simulink model "LPDs_single_agent_tech"  (R2023b)
settings: Solver=VariableStepAuto  StartTime=0.0  StopTime=24  FixedStep=0.005  RelTol=1e-6
undefined symbols (not defined in the file): battery_capacity_state_lower_limit, battery_capacity_state_upper_limit, battery_charge_power_state_lower_limit, battery_charge_power_state_upper_limit, battery_discharge_power_state_lower_limit, battery_discharge_power_state_upper_limit, battery_initial_capacity, battery_SOC_state_lower_limit, battery_SOC_state_upper_limit, EV_load_priority_factor, EV_load_rating, EV_load_state_lower_limit, EV_load_state_upper_limit, micro_grid_controller_power_state_lower_limit, micro_grid_controller_power_state_upper_limit, nano_grid_controller_power_rating, nano_grid_controller_power_state_lower_limit, nano_grid_controller_power_state_upper_limit, PV_power_rating, PV_power_state_lower_limit, PV_power_state_upper_limit, static_load_priority_factor, static_load_rating, static_load_state_lower_limit, static_load_state_upper_limit, sum_power_threshold_lower_limit, sum_power_threshold_upper_limit, TCL_load_priority_factor, TCL_load_rating, TCL_load_state_lower_limit, TCL_load_state_upper_limit, Wind_power_rating, Wind_power_state_lower_limit, Wind_power_state_upper_limit
libraries: spsStairGeneratorLib x13, simulink x7, slpidlib x2, rllib x2
(part 3 of 4)

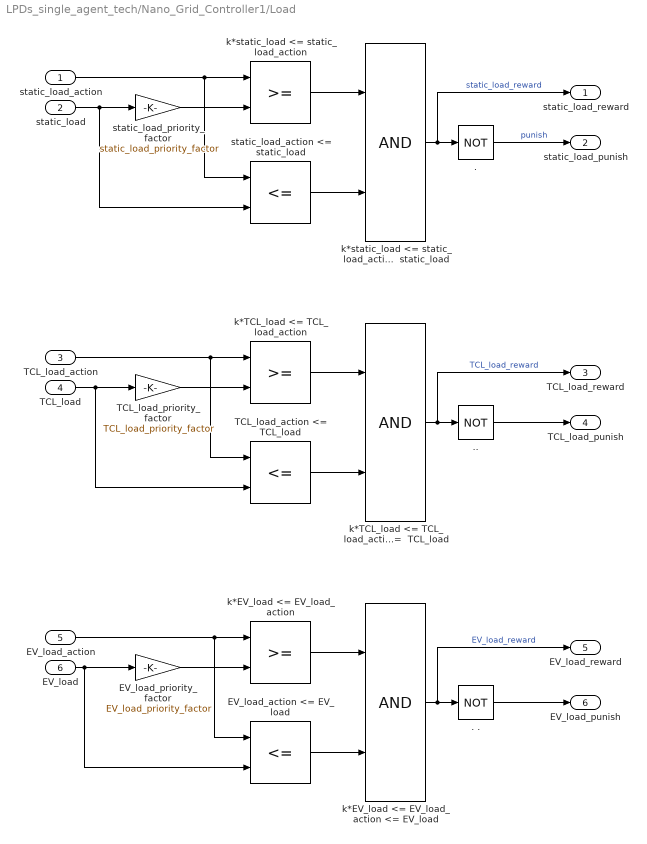
== system LPDs_single_agent_tech/Nano_Grid_Controller1/Load ==
  static_load_action : Inport
  static_load : Inport  Port=2
  TCL_load_action : Inport  Port=3
  TCL_load : Inport  Port=4
  EV_load_action : Inport  Port=5
  EV_load : Inport  Port=6
  . : Logic  Operator=NOT  IconShape=distinctive  AllPortsSameDT=off  OutDataTypeStr=boolean
  . . : Logic  Operator=NOT  IconShape=distinctive  AllPortsSameDT=off  OutDataTypeStr=boolean
  .. : Logic  Operator=NOT  IconShape=distinctive  AllPortsSameDT=off  OutDataTypeStr=boolean
  EV_load_action <= EV_load : RelationalOperator  Operator=<=  OutDataTypeStr=boolean  RndMeth=Simplest  InputSameDT=off
  EV_load_priority_factor : Gain  Gain=EV_load_priority_factor
  TCL_load_action <= TCL_load : RelationalOperator  Operator=<=  OutDataTypeStr=boolean  RndMeth=Simplest  InputSameDT=off
  TCL_load_priority_factor : Gain  Gain=TCL_load_priority_factor
  k*EV_load <= EV_load_action : RelationalOperator  OutDataTypeStr=boolean  RndMeth=Simplest  InputSameDT=off
  k*EV_load <= EV_load_action <= EV_load : Logic  IconShape=distinctive  AllPortsSameDT=off  OutDataTypeStr=boolean
  k*TCL_load <= TCL_load_action : RelationalOperator  OutDataTypeStr=boolean  RndMeth=Simplest  InputSameDT=off
  k*TCL_load <= TCL_load_action <=  TCL_load : Logic  IconShape=distinctive  AllPortsSameDT=off  OutDataTypeStr=boolean
  k*static_load <= static_load_action : RelationalOperator  OutDataTypeStr=boolean  RndMeth=Simplest  InputSameDT=off
  "k*static_load <= static_load_action <=  static_load " : Logic  IconShape=distinctive  AllPortsSameDT=off  OutDataTypeStr=boolean
  static_load_action <= static_load : RelationalOperator  Operator=<=  OutDataTypeStr=boolean  RndMeth=Simplest  InputSameDT=off
  static_load_priority_factor : Gain  Gain=static_load_priority_factor
  static_load_reward : Outport
  static_load_punish : Outport  Port=2
  TCL_load_reward : Outport  Port=3
  TCL_load_punish : Outport  Port=4
  EV_load_reward : Outport  Port=5
  EV_load_punish : Outport  Port=6
  wires:
  "k*static_load <= static_load_action <=  static_load "/1 -> static_load_reward/1, ./1  "static_load_reward"
  EV_load_priority_factor/1 -> k*EV_load <= EV_load_action/2
  EV_load_action <= EV_load/1 -> k*EV_load <= EV_load_action <= EV_load/2
  k*static_load <= static_load_action/1 -> "k*static_load <= static_load_action <=  static_load "/1
  k*TCL_load <= TCL_load_action <=  TCL_load/1 -> TCL_load_reward/1, ../1  "TCL_load_reward"
  k*EV_load <= EV_load_action <= EV_load/1 -> EV_load_reward/1, . ./1  "EV_load_reward"
  k*TCL_load <= TCL_load_action/1 -> k*TCL_load <= TCL_load_action <=  TCL_load/1
  static_load_action <= static_load/1 -> "k*static_load <= static_load_action <=  static_load "/2
  TCL_load_action <= TCL_load/1 -> k*TCL_load <= TCL_load_action <=  TCL_load/2
  EV_load_action/1 -> EV_load_action <= EV_load/1, k*EV_load <= EV_load_action/1
  static_load_priority_factor/1 -> k*static_load <= static_load_action/2
  TCL_load_priority_factor/1 -> k*TCL_load <= TCL_load_action/2
  k*EV_load <= EV_load_action/1 -> k*EV_load <= EV_load_action <= EV_load/1
  TCL_load/1 -> TCL_load_action <= TCL_load/2, TCL_load_priority_factor/1
  TCL_load_action/1 -> k*TCL_load <= TCL_load_action/1, TCL_load_action <= TCL_load/1
  static_load_action/1 -> k*static_load <= static_load_action/1, static_load_action <= static_load/1
  . ./1 -> EV_load_punish/1
  ../1 -> TCL_load_punish/1
  ./1 -> static_load_punish/1  "punish"
  static_load/1 -> static_load_action <= static_load/2, static_load_priority_factor/1
  EV_load/1 -> EV_load_action <= EV_load/2, EV_load_priority_factor/1

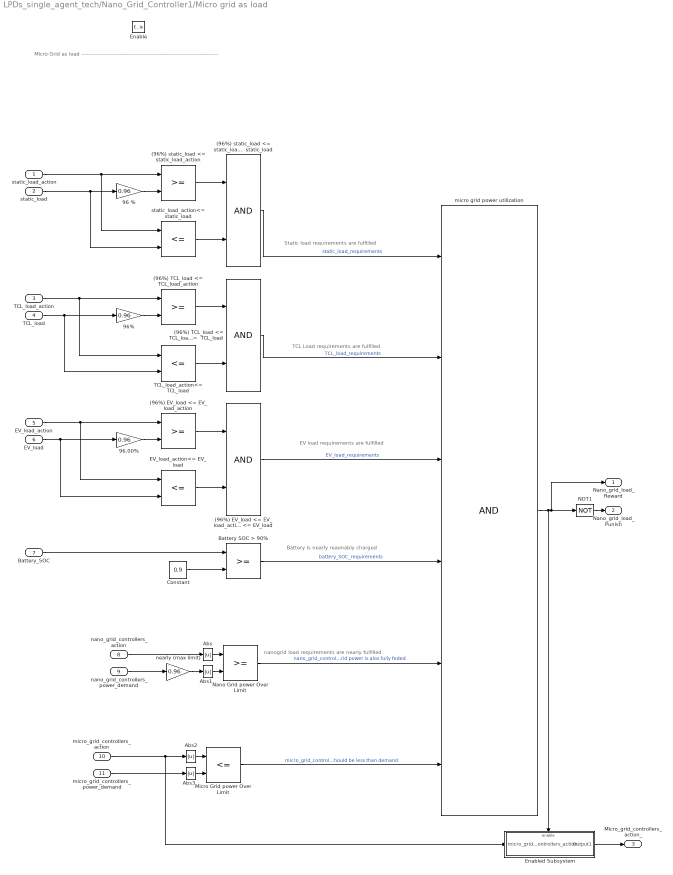
== system LPDs_single_agent_tech/Nano_Grid_Controller1/Micro grid as load ==
  note: Static load requirements are fulfilled
  note: Micro Grid as load
      | ----------------------------------------------------------------------------------
  note: TCL Load requirements are fulfilled
  note: EV load requirements are fulfilled
  note: Battery is nearly reaonably charged
  note: nanogrid load requirements are nearly fulfilled
  static_load_action : Inport
  static_load : Inport  Port=2
  TCL_load_action : Inport  Port=3
  TCL_load : Inport  Port=4
  EV_load_action : Inport  Port=5
  EV_load : Inport  Port=6
  Battery_SOC : Inport  Port=7
  nano_grid_controllers_action : Inport  Port=8
  nano_grid_controllers_power_demand : Inport  Port=9
  micro_grid_controllers_action : Inport  Port=10
  micro_grid_controllers_power_demand : Inport  Port=11
  Enable : EnablePort
  (96%) EV_load <= EV_load_action : RelationalOperator  OutDataTypeStr=boolean  RndMeth=Simplest  InputSameDT=off
  (96%) EV_load <= EV_load_action <= EV_load : Logic  IconShape=distinctive  AllPortsSameDT=off  OutDataTypeStr=boolean
  (96%) TCL_load <= TCL_load_action : RelationalOperator  OutDataTypeStr=boolean  RndMeth=Simplest  InputSameDT=off
  (96%) TCL_load <= TCL_load_action <=  TCL_load : Logic  IconShape=distinctive  AllPortsSameDT=off  OutDataTypeStr=boolean
  (96%) static_load <= static_load_action : RelationalOperator  OutDataTypeStr=boolean  RndMeth=Simplest  InputSameDT=off
  (96%) static_load <= static_load_action <=  static_load : Logic  IconShape=distinctive  AllPortsSameDT=off  OutDataTypeStr=boolean
  96 % : Gain  Gain=0.96
  96% : Gain  Gain=0.96
  96.00% : Gain  Gain=0.96
  Abs{,1..3} (4 alike) : Abs  SaturateOnIntegerOverflow=off
  Battery SOC > 90% : RelationalOperator  OutDataTypeStr=boolean  RndMeth=Simplest  InputSameDT=off
  Constant : Constant  Value=0.9
  EV_load_action<= EV_load : RelationalOperator  Operator=<=  OutDataTypeStr=boolean  RndMeth=Simplest  InputSameDT=off
  Enabled Subsystem : Subsystem  TreatAsAtomicUnit=on
  Micro Grid power Over Limit : RelationalOperator  Operator=<=  OutDataTypeStr=boolean  RndMeth=Simplest  InputSameDT=off
  NOT1 : Logic  Operator=NOT  Inputs=4  IconShape=distinctive  AllPortsSameDT=off  OutDataTypeStr=boolean
  Nano Grid power Over Limit : RelationalOperator  OutDataTypeStr=boolean  RndMeth=Simplest  InputSameDT=off
  TCL_load_action<= TCL_load : RelationalOperator  Operator=<=  OutDataTypeStr=boolean  RndMeth=Simplest  InputSameDT=off
  micro grid power utilization : Logic  Inputs=6  IconShape=distinctive  AllPortsSameDT=off  OutDataTypeStr=boolean
  nearly (max limit) : Gain  Gain=0.96
  static_load_action<= static_load : RelationalOperator  Operator=<=  OutDataTypeStr=boolean  RndMeth=Simplest  InputSameDT=off
  Nano_grid_load_Reward : Outport
  Nano_grid_load_Punish : Outport  Port=2
  Micro_grid_controllers_action_ : Outport  Port=3
  wires:
  (96%) TCL_load <= TCL_load_action <=  TCL_load/1 -> micro grid power utilization/2  "TCL_load_requirements"
  (96%) EV_load <= EV_load_action <= EV_load/1 -> micro grid power utilization/3  "EV_load_requirements"
  96%/1 -> (96%) TCL_load <= TCL_load_action/2
  TCL_load_action<= TCL_load/1 -> (96%) TCL_load <= TCL_load_action <=  TCL_load/2
  (96%) static_load <= static_load_action/1 -> (96%) static_load <= static_load_action <=  static_load/1
  TCL_load_action/1 -> TCL_load_action<= TCL_load/1, (96%) TCL_load <= TCL_load_action/1
  96 %/1 -> (96%) static_load <= static_load_action/2
  96.00%/1 -> (96%) EV_load <= EV_load_action/2
  (96%) EV_load <= EV_load_action/1 -> (96%) EV_load <= EV_load_action <= EV_load/1
  EV_load_action<= EV_load/1 -> (96%) EV_load <= EV_load_action <= EV_load/2
  static_load/1 -> static_load_action<= static_load/2, 96 %/1
  static_load_action<= static_load/1 -> (96%) static_load <= static_load_action <=  static_load/2
  EV_load/1 -> EV_load_action<= EV_load/2, 96.00%/1
  (96%) TCL_load <= TCL_load_action/1 -> (96%) TCL_load <= TCL_load_action <=  TCL_load/1
  Constant/1 -> Battery SOC > 90%/2
  static_load_action/1 -> static_load_action<= static_load/1, (96%) static_load <= static_load_action/1
  Battery SOC > 90%/1 -> micro grid power utilization/4  "battery_SOC_requirements"
  EV_load_action/1 -> EV_load_action<= EV_load/1, (96%) EV_load <= EV_load_action/1
  TCL_load/1 -> TCL_load_action<= TCL_load/2, 96%/1
  Battery_SOC/1 -> Battery SOC > 90%/1
  (96%) static_load <= static_load_action <=  static_load/1 -> micro grid power utilization/1  "static_load_requirements"
  Nano Grid power Over Limit/1 -> micro grid power utilization/5  "nano_grid_controllers_action >= 96% nano_grid_controllers_power_supply nano grid power is alos fully feded"
  nano_grid_controllers_power_demand/1 -> nearly (max limit)/1
  micro grid power utilization/1 -> NOT1/1, Nano_grid_load_Reward/1, Enabled Subsystem/Enable
  Enabled Subsystem/1(Output1) -> Micro_grid_controllers_action_/1
  NOT1/1 -> Nano_grid_load_Punish/1
  nano_grid_controllers_action/1 -> Abs/1
  Abs1/1 -> Nano Grid power Over Limit/2
  Abs/1 -> Nano Grid power Over Limit/1
  nearly (max limit)/1 -> Abs1/1
  Abs3/1 -> Micro Grid power Over Limit/2
  micro_grid_controllers_action/1 -> Enabled Subsystem/1(micro_grid_controllers_action), Abs2/1
  Abs2/1 -> Micro Grid power Over Limit/1
  Micro Grid power Over Limit/1 -> micro grid power utilization/6  "micro_grid_controllers_action >= micro_grid_controllers_power_supply micro grid feeding power should be less than demand"
  micro_grid_controllers_power_demand/1 -> Abs3/1

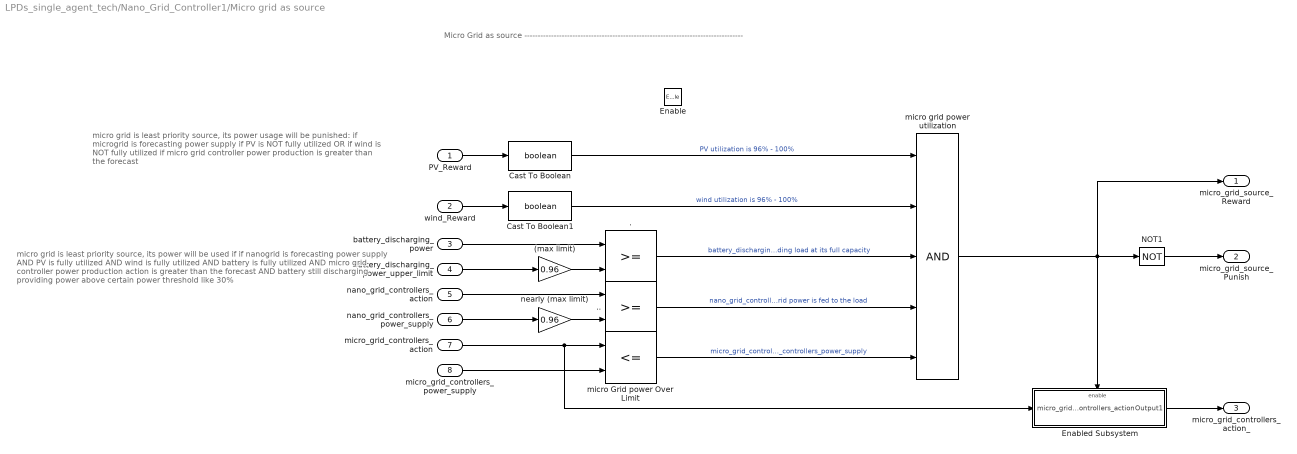
== system LPDs_single_agent_tech/Nano_Grid_Controller1/Micro grid as source ==
  note: Micro Grid as source
      | ----------------------------------------------------------------------------------
  note: micro grid is least priority source, its power usage will be punished:
      | if microgrid is forecasting power supply
      | if PV is NOT fully utilized OR
      | if wind is NOT fully utilized
      | if micro grid controller power production is greater than the forecast
  note: micro grid is least priority source, its power will be used if
      | if nanogrid is forecasting power supply
      | AND
      | PV is fully utilized
      | AND
      | wind is fully utilized
      | AND
      | battery is fully utilized
      | AND
      | micro grid controller power production action is greater than the forecast
      | AND
      | battery still discharging providing power above certain power threshold like 30%
  PV_Reward : Inport
  wind_Reward : Inport  Port=2
  battery_discharging_power : Inport  Port=3
  battery_discharging_power_upper_limit : Inport  Port=4
  nano_grid_controllers_action : Inport  Port=5
  nano_grid_controllers_power_supply : Inport  Port=6
  micro_grid_controllers_action : Inport  Port=7
  micro_grid_controllers_power_supply : Inport  Port=8
  Enable : EnablePort
  (max limit) : Gain  Gain=0.96
  . : RelationalOperator  OutDataTypeStr=boolean  RndMeth=Simplest  InputSameDT=off
  .. : RelationalOperator  OutDataTypeStr=boolean  RndMeth=Simplest  InputSameDT=off
  Cast To Boolean : DataTypeConversion  OutDataTypeStr=boolean  SaturateOnIntegerOverflow=off  RndMeth=Floor
  Cast To Boolean1 : DataTypeConversion  OutDataTypeStr=boolean  SaturateOnIntegerOverflow=off  RndMeth=Floor
  Enabled Subsystem : Subsystem  TreatAsAtomicUnit=on
  NOT1 : Logic  Operator=NOT  Inputs=4  IconShape=distinctive  AllPortsSameDT=off  OutDataTypeStr=boolean
  micro Grid power Over Limit : RelationalOperator  Operator=<=  OutDataTypeStr=boolean  RndMeth=Simplest  InputSameDT=off
  micro grid power utilization : Logic  Inputs=5  IconShape=distinctive  AllPortsSameDT=off  OutDataTypeStr=boolean
  nearly (max limit) : Gain  Gain=0.96
  micro_grid_source_Reward : Outport
  micro_grid_source_Punish : Outport  Port=2
  micro_grid_controllers_action_ : Outport  Port=3
  wires:
  wind_Reward/1 -> Cast To Boolean1/1
  ../1 -> micro grid power utilization/4  "nano_grid_controllers_action >= 96% nano_grid_controllers_power_supply all of the nanogrid power is fed to the load"
  PV_Reward/1 -> Cast To Boolean/1
  nano_grid_controllers_action/1 -> ../1
  micro grid power utilization/1 -> micro_grid_source_Reward/1, NOT1/1, Enabled Subsystem/Enable
  nano_grid_controllers_power_supply/1 -> nearly (max limit)/1
  Enabled Subsystem/1(Output1) -> micro_grid_controllers_action_/1
  NOT1/1 -> micro_grid_source_Punish/1
  Cast To Boolean/1 -> micro grid power utilization/1  "PV utilization is 96% - 100%"
  Cast To Boolean1/1 -> micro grid power utilization/2  "wind utilization is 96% - 100%"
  battery_discharging_power/1 -> ./1
  ./1 -> micro grid power utilization/3  "battery_discharging_power >= 96 % of max limit battery is feeding load at its full capacity"
  battery_discharging_power_upper_limit/1 -> (max limit)/1
  (max limit)/1 -> ./2
  nearly (max limit)/1 -> ../2
  micro_grid_controllers_power_supply/1 -> micro Grid power Over Limit/2
  micro_grid_controllers_action/1 -> micro Grid power Over Limit/1, Enabled Subsystem/1(micro_grid_controllers_action)
  micro Grid power Over Limit/1 -> micro grid power utilization/5  "micro_grid_controllers_action <= micro_grid_controllers_power_supply"

== system LPDs_single_agent_tech/Nano_Grid_Controller1/PV-System ==
  note: PV_power_current_capacity
  note: 0.96*P_pv < P_pv (t) < P_pv_max
  PV1_power : Inport
  " 0.96*P_pv < P_PV (t)" : RelationalOperator  OutDataTypeStr=boolean  RndMeth=Simplest  InputSameDT=off
  " P_PV (t) <= P_PV_max" : RelationalOperator  Operator=<=  OutDataTypeStr=boolean  RndMeth=Simplest  InputSameDT=off
  Gain1 : Gain  Gain=0.96
  NOT1 : Logic  Operator=NOT  Inputs=4  IconShape=distinctive  AllPortsSameDT=off  OutDataTypeStr=boolean
  PID Controller : slpidlib/PID Controller  Controller=PID  Form=Parallel  TimeDomain=Continuous-time  UseExternalTs=off  SampleTime=-1  IntegratorMethod=Forward Euler  FilterMethod=Forward Euler  ControllerParametersSource=internal  P=15.7600865897305  I=69739.5529413598  UseKiTs=off  D=0.000244643612586244  N=25330.5649262246  UseFilter=on  TunerSelectOption=Transfer Function Based (PID Tuner App)  InitialConditionSource=internal  InitialConditionForIntegrator=0  InitialConditionForFilter=0  DifferentiatorICPrevScaledInput=0  ExternalReset=none  TrackingMode=off  Kt=1  LimitOutput=off  SatLimitsSource=internal  UpperSaturationLimit=inf  LowerSaturationLimit=-inf  LinearizeAsGain=on  AntiWindupMode=none  Kb=1  LimitIntegrator=off  UpperIntegratorSaturationLimit=inf  LowerIntegratorSaturationLimit=-inf  POutMin=[]  POutMax=[]  IOutMin=[]  IOutMax=[]  DOutMin=[]  DOutMax=[]  NOutMin=[]  NOutMax=[]  SumOutMin=[]  SumOutMax=[]  SaturationOutMin=[]  SaturationOutMax=[]  PParamMin=[]  PParamMax=[]  IParamMin=[]  IParamMax=[]  DParamMin=[]  DParamMax=[]  NParamMin=[]  NParamMax=[]  KbParamMin=[]  KbParamMax=[]  KtParamMin=[]  KtParamMax=[]  KbOutMin=[]  KbOutMax=[]  KtOutMin=[]  KtOutMax=[]  IntegratorOutMin=[]  IntegratorOutMax=[]  FilterOutMin=[]  FilterOutMax=[]  SumI1OutMin=[]  SumI1OutMax=[]  SumI2OutMin=[]  SumI2OutMax=[]  SumI3OutMin=[]  SumI3OutMax=[]  SumI4OutMin=[]  SumI4OutMax=[]  SumDOutMin=[]  SumDOutMax=[]  DifferentiatorOutMin=[]  DifferentiatorOutMax=[]  FilterDiffOutCoefMin=[]  FilterDiffOutCoefMax=[]  ReciprocalOutMin=[]  ReciprocalOutMax=[]  SumDenOutMin=[]  SumDenOutMax=[]  SumNumOutMin=[]  SumNumOutMax=[]  DivideOutMin=[]  DivideOutMax=[]  UdiffTsProdOutMin=[]  UdiffTsProdOutMax=[]  NTsProdOutMin=[]  NTsProdOutMax=[]  UintegralTsProdOutMin=[]  UintegralTsProdOutMax=[]  UngainTsProdOutMin=[]  UngainTsProdOutMax=[]  ClampingZeroOutDataTypeStr=Inherit: Inherit via back propagation  ClampingZeroOutMin=[]  ClampingZeroOutMax=[]  FilterDenConstantOutDataTypeStr=Inherit: Inherit via back propagation  FilterDenConstantOutMin=[]  FilterDenConstantOutMax=[]  PCopyOutDataTypeStr=Inherit: Inherit via back propagation  PCopyOutMin=[]  PCopyOutMax=[]  NCopyOutDataTypeStr=Inherit: Inherit via back propagation  NCopyOutMin=[]  NCopyOutMax=[]  IntegratorContinuousStateAttributes=''  IntegratorStateMustResolveToSignalObject=off  IntegratorRTWStateStorageClass=Auto  FilterContinuousStateAttributes=''  FilterStateMustResolveToSignalObject=off  FilterRTWStateStorageClass=Auto  ParallelPVariant=InternalParameters  IdealPVariant=Disabled  IVariant=InternalParameters  DVariant=InternalParameters  IntegratorVariant=Continuous  SatVariant=Disabled  AWVariant=Passthrough  PCopyVariant=Disabled  TRVariant=Disabled  FdbkBlocksVariant=Forward  IdealPFdbkVariant=Disabled  SatFdbkVariant=Disabled  DerivativeFilterVariant=ContFilter  NVariant=InternalParameters  NCopyVariant=Disabled  FilterICVariant=InternalICsFilter  IntegratorICVariant=InternalICs  ExternalResetVariant=Disabled  TRSumVariant=Passthrough  SumFdbkVariant=Disabled  SumVariant=Sum_PID  TsampFilterVariant=InternalTs  TsampNgainVariant=Passthrough  TsampIntegralVariant=Disabled_SignalSpec  ExternalSaturationOutDataTypeStr=Inherit: Same as second input
  PV power utilization : Logic  IconShape=distinctive  AllPortsSameDT=off  OutDataTypeStr=boolean
  Scope : Scope  NumInputPorts=2
  Scope1 : Scope
  Subsystem : Subsystem
  Sum2 : Sum  Inputs=|+-
  Transfer Fcn : TransferFcn  Denominator=[0.001 1]
  PV1_power_actions : Outport
  PV_Reward : Outport  Port=2
  PV_punish : Outport  Port=3
  wires:
  " 0.96*P_pv < P_PV (t)"/1 -> PV power utilization/1
  PV power utilization/1 -> PV_Reward/1, Scope1/1, NOT1/1
  " P_PV (t) <= P_PV_max"/1 -> PV power utilization/2
  Gain1/1 -> " 0.96*P_pv < P_PV (t)"/2
  NOT1/1 -> PV_punish/1, Subsystem/Enable
  PV1_power/1 -> Scope/1, Gain1/1, " P_PV (t) <= P_PV_max"/2, Sum2/1
  Transfer Fcn/1 -> Sum2/2, " P_PV (t) <= P_PV_max"/1, " 0.96*P_pv < P_PV (t)"/1, Scope/2, PV1_power_actions/1
  PID Controller/1 -> Transfer Fcn/1
  Subsystem/1(y) -> PID Controller/1
  Sum2/1 -> Subsystem/1(u)  "error"

== system LPDs_single_agent_tech/Nano_Grid_Controller1/Subsystem1 ==
  observation : Inport
  reward : Inport  Port=2
  isdone : Inport  Port=3
  Demux20 : Demux  Outputs=8
  Memory2 : Memory
  RL Agent2 : rllib/RL Agent  Commented=on  Agent=agent1  ExternalActionAsInput=off  ProvideLastAction=off  ProvideCumRwd=off  TreatAsDirectFeedthrough=on  UseStrictObservationDataTypes=off
  Out1 : Outport
  Out2 : Outport  Port=2
  Out3 : Outport  Port=3
  Out4 : Outport  Port=4
  Out5 : Outport  Port=5
  Out6 : Outport  Port=6
  Out7 : Outport  Port=7
  Out8 : Outport  Port=8
  wires:
  Demux20/2 -> Out2/1
  Demux20/4 -> Out4/1
  Demux20/8 -> Out8/1
  Demux20/7 -> Out7/1
  Memory2/1 -> Demux20/1
  Demux20/6 -> Out6/1
  RL Agent2/1 -> Memory2/1
  Demux20/1 -> Out1/1
  Demux20/3 -> Out3/1
  isdone/1 -> RL Agent2/3
  Demux20/5 -> Out5/1
  reward/1 -> RL Agent2/2
  observation/1 -> RL Agent2/1

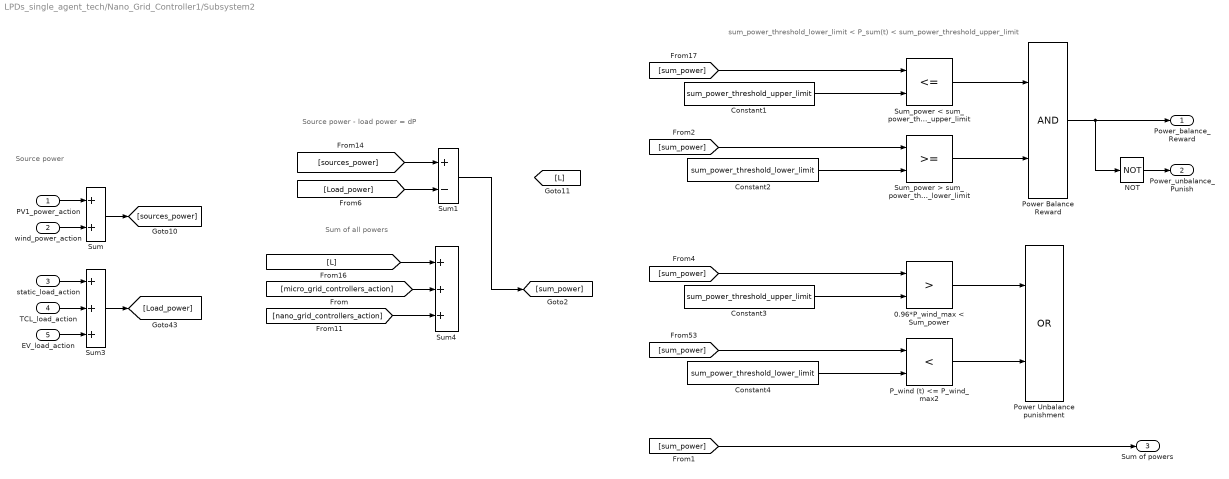
== system LPDs_single_agent_tech/Nano_Grid_Controller1/Subsystem2 ==
  note: sum_power_threshold_lower_limit < P_sum(t) < sum_power_threshold_upper_limit
  note: Source power - load power = dP
  note: Sum of all powers
  note: Source power
  PV1_power_action : Inport
  wind_power_action : Inport  Port=2
  static_load_action : Inport  Port=3
  TCL_load_action : Inport  Port=4
  EV_load_action : Inport  Port=5
  "  Sum_power < sum_power_threshold_upper_limit" : RelationalOperator  Operator=<=  OutDataTypeStr=boolean  RndMeth=Simplest  InputSameDT=off
  "  Sum_power > sum_power_threshold_lower_limit" : RelationalOperator  OutDataTypeStr=boolean  RndMeth=Simplest  InputSameDT=off
  " 0.96*P_wind_max < Sum_power" : RelationalOperator  Operator=>  OutDataTypeStr=boolean  RndMeth=Simplest  InputSameDT=off
  " P_wind (t) <= P_wind_max2" : RelationalOperator  Operator=<  OutDataTypeStr=boolean  RndMeth=Simplest  InputSameDT=off
  Constant1 : Constant  Value=sum_power_threshold_upper_limit
  Constant2 : Constant  Value=sum_power_threshold_lower_limit
  Constant3 : Constant  Value=sum_power_threshold_upper_limit
  Constant4 : Constant  Value=sum_power_threshold_lower_limit
  NOT : Logic  Operator=NOT  IconShape=distinctive  AllPortsSameDT=off  OutDataTypeStr=boolean
  Power Balance Reward : Logic  IconShape=distinctive  AllPortsSameDT=off  OutDataTypeStr=boolean
  Power Unbalance punishment : Logic  Operator=OR  IconShape=distinctive  AllPortsSameDT=off  OutDataTypeStr=boolean
  Sum : Sum
  Sum1 : Sum  Inputs=+-
  Sum3 : Sum  Inputs=+++
  Sum4 : Sum  Inputs=+++
  Power_balance_Reward : Outport
  Power_unbalance_Punish : Outport  Port=2
  Sum of powers : Outport  Port=3
  wires:
  [Load_power] -> Sum1/2
  Sum3/1 -> [Load_power]
  NOT/1 -> Power_unbalance_Punish/1
  [sum_power] -> " 0.96*P_wind_max < Sum_power"/1
  Sum1/1 -> [sum_power]
  TCL_load_action/1 -> Sum3/2
  " 0.96*P_wind_max < Sum_power"/1 -> Power Unbalance punishment/1
  [sum_power] -> "  Sum_power < sum_power_threshold_upper_limit"/1
  " P_wind (t) <= P_wind_max2"/1 -> Power Unbalance punishment/2
  Sum/1 -> [sources_power]
  "  Sum_power < sum_power_threshold_upper_limit"/1 -> Power Balance Reward/1
  ? -> [L]
  [sources_power] -> Sum1/1
  [sum_power] -> " P_wind (t) <= P_wind_max2"/1
  EV_load_action/1 -> Sum3/3
  "  Sum_power > sum_power_threshold_lower_limit"/1 -> Power Balance Reward/2
  [L] -> Sum4/1
  wind_power_action/1 -> Sum/2
  Constant1/1 -> "  Sum_power < sum_power_threshold_upper_limit"/2
  Constant2/1 -> "  Sum_power > sum_power_threshold_lower_limit"/2
  Constant3/1 -> " 0.96*P_wind_max < Sum_power"/2
  Constant4/1 -> " P_wind (t) <= P_wind_max2"/2
  [sum_power] -> "  Sum_power > sum_power_threshold_lower_limit"/1
  [micro_grid_controllers_action] -> Sum4/2
  [nano_grid_controllers_action] -> Sum4/3
  Power Balance Reward/1 -> NOT/1, Power_balance_Reward/1
  static_load_action/1 -> Sum3/1
  PV1_power_action/1 -> Sum/1
  [sum_power] -> Sum of powers/1

== system LPDs_single_agent_tech/Nano_Grid_Controller1/Wind power utilization ==
  note: 0.9*P_wind_max < P_wind (t) < P_wind_max
  note: wind_power_current_capacity
  Wind_power : Inport
  " 0.96*P_wind_max < P_wind (t)" : RelationalOperator  OutDataTypeStr=boolean  RndMeth=Simplest  InputSameDT=off
  " P_wind (t) <= P_wind_max" : RelationalOperator  Operator=<=  OutDataTypeStr=boolean  RndMeth=Simplest  InputSameDT=off
  Gain1 : Gain  Gain=0.9
  NOT2 : Logic  Operator=NOT  Inputs=4  IconShape=distinctive  AllPortsSameDT=off  OutDataTypeStr=boolean
  PID Controller : slpidlib/PID Controller  Controller=PID  Form=Parallel  TimeDomain=Continuous-time  UseExternalTs=off  SampleTime=-1  IntegratorMethod=Forward Euler  FilterMethod=Forward Euler  ControllerParametersSource=internal  P=15.7600865897305  I=69739.5529413598  UseKiTs=off  D=0.000244643612586244  N=25330.5649262246  UseFilter=on  TunerSelectOption=Transfer Function Based (PID Tuner App)  InitialConditionSource=internal  InitialConditionForIntegrator=0  InitialConditionForFilter=0  DifferentiatorICPrevScaledInput=0  ExternalReset=none  TrackingMode=off  Kt=1  LimitOutput=off  SatLimitsSource=internal  UpperSaturationLimit=inf  LowerSaturationLimit=-inf  LinearizeAsGain=on  AntiWindupMode=none  Kb=1  LimitIntegrator=off  UpperIntegratorSaturationLimit=inf  LowerIntegratorSaturationLimit=-inf  POutMin=[]  POutMax=[]  IOutMin=[]  IOutMax=[]  DOutMin=[]  DOutMax=[]  NOutMin=[]  NOutMax=[]  SumOutMin=[]  SumOutMax=[]  SaturationOutMin=[]  SaturationOutMax=[]  PParamMin=[]  PParamMax=[]  IParamMin=[]  IParamMax=[]  DParamMin=[]  DParamMax=[]  NParamMin=[]  NParamMax=[]  KbParamMin=[]  KbParamMax=[]  KtParamMin=[]  KtParamMax=[]  KbOutMin=[]  KbOutMax=[]  KtOutMin=[]  KtOutMax=[]  IntegratorOutMin=[]  IntegratorOutMax=[]  FilterOutMin=[]  FilterOutMax=[]  SumI1OutMin=[]  SumI1OutMax=[]  SumI2OutMin=[]  SumI2OutMax=[]  SumI3OutMin=[]  SumI3OutMax=[]  SumI4OutMin=[]  SumI4OutMax=[]  SumDOutMin=[]  SumDOutMax=[]  DifferentiatorOutMin=[]  DifferentiatorOutMax=[]  FilterDiffOutCoefMin=[]  FilterDiffOutCoefMax=[]  ReciprocalOutMin=[]  ReciprocalOutMax=[]  SumDenOutMin=[]  SumDenOutMax=[]  SumNumOutMin=[]  SumNumOutMax=[]  DivideOutMin=[]  DivideOutMax=[]  UdiffTsProdOutMin=[]  UdiffTsProdOutMax=[]  NTsProdOutMin=[]  NTsProdOutMax=[]  UintegralTsProdOutMin=[]  UintegralTsProdOutMax=[]  UngainTsProdOutMin=[]  UngainTsProdOutMax=[]  ClampingZeroOutDataTypeStr=Inherit: Inherit via back propagation  ClampingZeroOutMin=[]  ClampingZeroOutMax=[]  FilterDenConstantOutDataTypeStr=Inherit: Inherit via back propagation  FilterDenConstantOutMin=[]  FilterDenConstantOutMax=[]  PCopyOutDataTypeStr=Inherit: Inherit via back propagation  PCopyOutMin=[]  PCopyOutMax=[]  NCopyOutDataTypeStr=Inherit: Inherit via back propagation  NCopyOutMin=[]  NCopyOutMax=[]  IntegratorContinuousStateAttributes=''  IntegratorStateMustResolveToSignalObject=off  IntegratorRTWStateStorageClass=Auto  FilterContinuousStateAttributes=''  FilterStateMustResolveToSignalObject=off  FilterRTWStateStorageClass=Auto  ParallelPVariant=InternalParameters  IdealPVariant=Disabled  IVariant=InternalParameters  DVariant=InternalParameters  IntegratorVariant=Continuous  SatVariant=Disabled  AWVariant=Passthrough  PCopyVariant=Disabled  TRVariant=Disabled  FdbkBlocksVariant=Forward  IdealPFdbkVariant=Disabled  SatFdbkVariant=Disabled  DerivativeFilterVariant=ContFilter  NVariant=InternalParameters  NCopyVariant=Disabled  FilterICVariant=InternalICsFilter  IntegratorICVariant=InternalICs  ExternalResetVariant=Disabled  TRSumVariant=Passthrough  SumFdbkVariant=Disabled  SumVariant=Sum_PID  TsampFilterVariant=InternalTs  TsampNgainVariant=Passthrough  TsampIntegralVariant=Disabled_SignalSpec  ExternalSaturationOutDataTypeStr=Inherit: Same as second input
  Scope : Scope  NumInputPorts=2
  Scope1 : Scope
  Subsystem : Subsystem
  Sum2 : Sum  Inputs=|+-
  Transfer Fcn : TransferFcn  Denominator=[0.001 1]
  Wind power utilization : Logic  IconShape=distinctive  AllPortsSameDT=off  OutDataTypeStr=boolean
  Wind_power_actions : Outport
  Wind_Reward : Outport  Port=2
  Wind_punish : Outport  Port=3
  wires:
  Subsystem/1(y) -> PID Controller/1
  PID Controller/1 -> Transfer Fcn/1
  Transfer Fcn/1 -> Scope/2, " P_wind (t) <= P_wind_max"/1, " 0.96*P_wind_max < P_wind (t)"/1, Sum2/2, Wind_power_actions/1
  Wind_power/1 -> Scope/1, Gain1/1, " P_wind (t) <= P_wind_max"/2, Sum2/1
  Sum2/1 -> Subsystem/1(u)  "error"
  Wind power utilization/1 -> Wind_Reward/1, Scope1/1, NOT2/1
  NOT2/1 -> Wind_punish/1, Subsystem/Enable
  " 0.96*P_wind_max < P_wind (t)"/1 -> Wind power utilization/1
  " P_wind (t) <= P_wind_max"/1 -> Wind power utilization/2
  Gain1/1 -> " 0.96*P_wind_max < P_wind (t)"/2

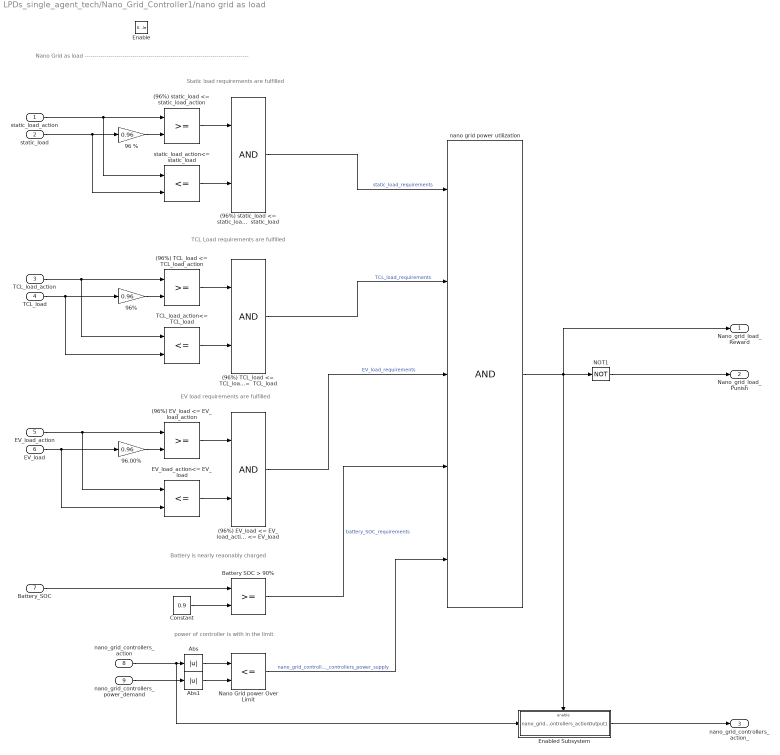
== system LPDs_single_agent_tech/Nano_Grid_Controller1/nano grid as load ==
  note: Static load requirements are fulfilled
  note: Nano Grid as load
      | ----------------------------------------------------------------------------------
  note: TCL Load requirements are fulfilled
  note: EV load requirements are fulfilled
  note: Battery is nearly reaonably charged
  note: power of controller is with in the limit
  static_load_action : Inport
  static_load : Inport  Port=2
  TCL_load_action : Inport  Port=3
  TCL_load : Inport  Port=4
  EV_load_action : Inport  Port=5
  EV_load : Inport  Port=6
  Battery_SOC : Inport  Port=7
  nano_grid_controllers_action : Inport  Port=8
  nano_grid_controllers_power_demand : Inport  Port=9
  Enable : EnablePort
  (96%) EV_load <= EV_load_action : RelationalOperator  OutDataTypeStr=boolean  RndMeth=Simplest  InputSameDT=off
  (96%) EV_load <= EV_load_action <= EV_load : Logic  IconShape=distinctive  AllPortsSameDT=off  OutDataTypeStr=boolean
  (96%) TCL_load <= TCL_load_action : RelationalOperator  OutDataTypeStr=boolean  RndMeth=Simplest  InputSameDT=off
  (96%) TCL_load <= TCL_load_action <=  TCL_load : Logic  IconShape=distinctive  AllPortsSameDT=off  OutDataTypeStr=boolean
  (96%) static_load <= static_load_action : RelationalOperator  OutDataTypeStr=boolean  RndMeth=Simplest  InputSameDT=off
  (96%) static_load <= static_load_action <=  static_load : Logic  IconShape=distinctive  AllPortsSameDT=off  OutDataTypeStr=boolean
  96 % : Gain  Gain=0.96
  96% : Gain  Gain=0.96
  96.00% : Gain  Gain=0.96
  Abs : Abs  SaturateOnIntegerOverflow=off
  Abs1 : Abs  SaturateOnIntegerOverflow=off
  Battery SOC > 90% : RelationalOperator  OutDataTypeStr=boolean  RndMeth=Simplest  InputSameDT=off
  Constant : Constant  Value=0.9
  EV_load_action<= EV_load : RelationalOperator  Operator=<=  OutDataTypeStr=boolean  RndMeth=Simplest  InputSameDT=off
  Enabled Subsystem : Subsystem  TreatAsAtomicUnit=on
  NOT1 : Logic  Operator=NOT  Inputs=4  IconShape=distinctive  AllPortsSameDT=off  OutDataTypeStr=boolean
  Nano Grid power Over Limit : RelationalOperator  Operator=<=  OutDataTypeStr=boolean  RndMeth=Simplest  InputSameDT=off
  TCL_load_action<= TCL_load : RelationalOperator  Operator=<=  OutDataTypeStr=boolean  RndMeth=Simplest  InputSameDT=off
  nano grid power utilization : Logic  Inputs=5  IconShape=distinctive  AllPortsSameDT=off  OutDataTypeStr=boolean
  static_load_action<= static_load : RelationalOperator  Operator=<=  OutDataTypeStr=boolean  RndMeth=Simplest  InputSameDT=off
  Nano_grid_load_Reward : Outport
  Nano_grid_load_Punish : Outport  Port=2
  nano_grid_controllers_action_ : Outport  Port=3
  wires:
  (96%) TCL_load <= TCL_load_action <=  TCL_load/1 -> nano grid power utilization/2  "TCL_load_requirements"
  (96%) EV_load <= EV_load_action <= EV_load/1 -> nano grid power utilization/3  "EV_load_requirements"
  96%/1 -> (96%) TCL_load <= TCL_load_action/2
  TCL_load_action<= TCL_load/1 -> (96%) TCL_load <= TCL_load_action <=  TCL_load/2
  (96%) static_load <= static_load_action/1 -> (96%) static_load <= static_load_action <=  static_load/1
  TCL_load_action/1 -> TCL_load_action<= TCL_load/1, (96%) TCL_load <= TCL_load_action/1
  96 %/1 -> (96%) static_load <= static_load_action/2
  96.00%/1 -> (96%) EV_load <= EV_load_action/2
  (96%) EV_load <= EV_load_action/1 -> (96%) EV_load <= EV_load_action <= EV_load/1
  EV_load_action<= EV_load/1 -> (96%) EV_load <= EV_load_action <= EV_load/2
  static_load/1 -> static_load_action<= static_load/2, 96 %/1
  static_load_action<= static_load/1 -> (96%) static_load <= static_load_action <=  static_load/2
  EV_load/1 -> EV_load_action<= EV_load/2, 96.00%/1
  (96%) TCL_load <= TCL_load_action/1 -> (96%) TCL_load <= TCL_load_action <=  TCL_load/1
  Constant/1 -> Battery SOC > 90%/2
  static_load_action/1 -> static_load_action<= static_load/1, (96%) static_load <= static_load_action/1
  Battery SOC > 90%/1 -> nano grid power utilization/4  "battery_SOC_requirements"
  EV_load_action/1 -> EV_load_action<= EV_load/1, (96%) EV_load <= EV_load_action/1
  TCL_load/1 -> TCL_load_action<= TCL_load/2, 96%/1
  Battery_SOC/1 -> Battery SOC > 90%/1
  (96%) static_load <= static_load_action <=  static_load/1 -> nano grid power utilization/1  "static_load_requirements"
  Nano Grid power Over Limit/1 -> nano grid power utilization/5  "nano_grid_controllers_action <= nano_grid_controllers_power_supply"
  nano_grid_controllers_power_demand/1 -> Abs1/1
  nano grid power utilization/1 -> NOT1/1, Nano_grid_load_Reward/1, Enabled Subsystem/Enable
  Enabled Subsystem/1(Output1) -> nano_grid_controllers_action_/1
  NOT1/1 -> Nano_grid_load_Punish/1
  nano_grid_controllers_action/1 -> Abs/1, Enabled Subsystem/1(nano_grid_controllers_action)
  Abs1/1 -> Nano Grid power Over Limit/2
  Abs/1 -> Nano Grid power Over Limit/1

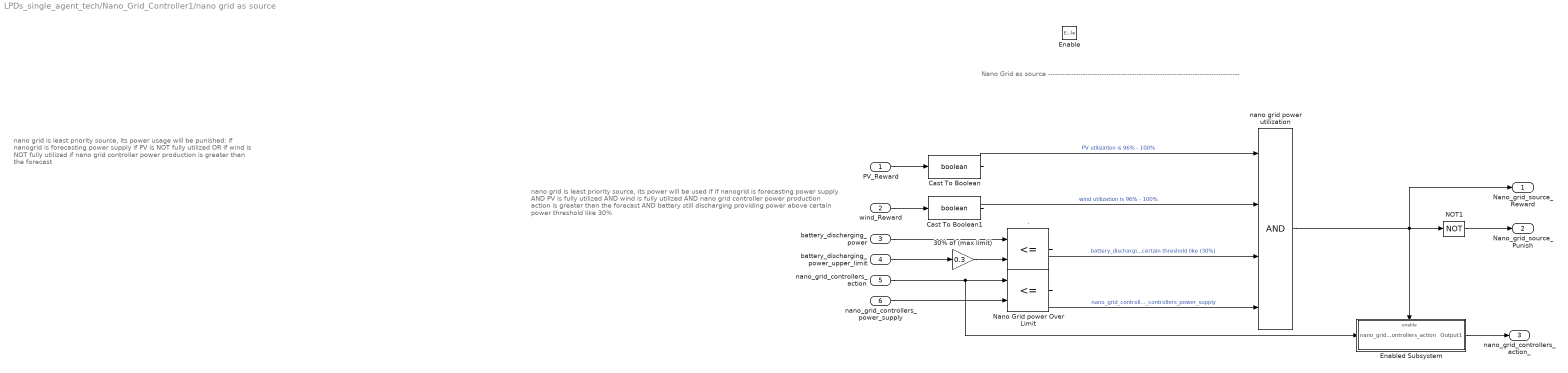
== system LPDs_single_agent_tech/Nano_Grid_Controller1/nano grid as source ==
  note: Nano Grid as source
      | ----------------------------------------------------------------------------------
  note: nano grid is least priority source, its power usage will be punished:
      | if nanogrid is forecasting power supply
      | if PV is NOT fully utilized OR
      | if wind is NOT fully utilized
      | if nano grid controller power production is greater than the forecast
  note: nano grid is least priority source, its power will be used if
      | if nanogrid is forecasting power supply
      | AND
      | PV is fully utilized
      | AND
      | wind is fully utilized
      | AND
      | nano grid controller power production action is greater than the forecast
      | AND
      | battery still discharging providing power above certain power threshold like 30%
  PV_Reward : Inport
  wind_Reward : Inport  Port=2
  battery_discharging_power : Inport  Port=3
  battery_discharging_power_upper_limit : Inport  Port=4
  nano_grid_controllers_action : Inport  Port=5
  nano_grid_controllers_power_supply : Inport  Port=6
  Enable : EnablePort
  . : RelationalOperator  Operator=<=  OutDataTypeStr=boolean  RndMeth=Simplest  InputSameDT=off
  30% of (max limit) : Gain  Gain=0.3
  Cast To Boolean : DataTypeConversion  OutDataTypeStr=boolean  SaturateOnIntegerOverflow=off  RndMeth=Floor
  Cast To Boolean1 : DataTypeConversion  OutDataTypeStr=boolean  SaturateOnIntegerOverflow=off  RndMeth=Floor
  Enabled Subsystem : Subsystem  TreatAsAtomicUnit=on
  NOT1 : Logic  Operator=NOT  Inputs=4  IconShape=distinctive  AllPortsSameDT=off  OutDataTypeStr=boolean
  Nano Grid power Over Limit : RelationalOperator  Operator=<=  OutDataTypeStr=boolean  RndMeth=Simplest  InputSameDT=off
  nano grid power utilization : Logic  Inputs=4  IconShape=distinctive  AllPortsSameDT=off  OutDataTypeStr=boolean
  Nano_grid_source_Reward : Outport
  Nano_grid_source_Punish : Outport  Port=2
  nano_grid_controllers_action_ : Outport  Port=3
  wires:
  wind_Reward/1 -> Cast To Boolean1/1
  Nano Grid power Over Limit/1 -> nano grid power utilization/4  "nano_grid_controllers_action <= nano_grid_controllers_power_supply"
  PV_Reward/1 -> Cast To Boolean/1
  nano_grid_controllers_action/1 -> Nano Grid power Over Limit/1, Enabled Subsystem/1(nano_grid_controllers_action)
  nano grid power utilization/1 -> Nano_grid_source_Reward/1, NOT1/1, Enabled Subsystem/Enable
  nano_grid_controllers_power_supply/1 -> Nano Grid power Over Limit/2
  Enabled Subsystem/1(Output1) -> nano_grid_controllers_action_/1
  NOT1/1 -> Nano_grid_source_Punish/1
  Cast To Boolean/1 -> nano grid power utilization/1  "PV utilization is 96% - 100%"
  Cast To Boolean1/1 -> nano grid power utilization/2  "wind utilization is 96% - 100%"
  battery_discharging_power/1 -> ./1
  ./1 -> nano grid power utilization/3  "battery_discharging_power <= 30 % of max limit battery is discharging above certain threshold like (30%)"
  battery_discharging_power_upper_limit/1 -> 30% of (max limit)/1
  30% of (max limit)/1 -> ./2

== system LPDs_single_agent_tech/Nano_Grid_Controller1/Micro grid as load/Enabled Subsystem ==
  micro_grid_controllers_action : Inport
  Enable : EnablePort
  Output1 : Outport
  wires:
  micro_grid_controllers_action/1 -> Output1/1

== system LPDs_single_agent_tech/Nano_Grid_Controller1/Micro grid as source/Enabled Subsystem ==
  micro_grid_controllers_action : Inport
  Enable : EnablePort
  Output1 : Outport
  wires:
  micro_grid_controllers_action/1 -> Output1/1

== system LPDs_single_agent_tech/Nano_Grid_Controller1/PV-System/Subsystem ==
  u : Inport
  Enable : EnablePort
  y : Outport
  wires:
  u/1 -> y/1

== system LPDs_single_agent_tech/Nano_Grid_Controller1/Wind power utilization/Subsystem ==
  u : Inport
  Enable : EnablePort
  y : Outport
  wires:
  u/1 -> y/1

== system LPDs_single_agent_tech/Nano_Grid_Controller1/nano grid as load/Enabled Subsystem ==
  nano_grid_controllers_action : Inport
  Enable : EnablePort
  Output1 : Outport
  wires:
  nano_grid_controllers_action/1 -> Output1/1

== system LPDs_single_agent_tech/Nano_Grid_Controller1/nano grid as source/Enabled Subsystem ==
  nano_grid_controllers_action : Inport
  Enable : EnablePort
  Output1 : Outport
  wires:
  nano_grid_controllers_action/1 -> Output1/1
